simulink model "test"  (R2018a)
settings: Solver=VariableStepAuto  StartTime=0.0  StopTime=50  RelTol=1e-3
values from neighbouring files (symbols this model uses):
  A = [0 0 0 0 1 0 0 0 0 2.100456621 0 36.0401472471 ... (16 elements, 4x4)]    [optimal_a1.mat]    (also in optimal_a2.mat; optimal_b1.mat; optimal_c1.mat; optimal_c3.mat)
  B = [0 0.931879601156 0 2.82216717491]    [optimal_a1.mat]    (also in optimal_a2.mat; optimal_b1.mat; optimal_c1.mat; optimal_c3.mat)
  C = [1  0  0  0; 0  0  1  0]    [optimal_a1.mat]    (also in optimal_a2.mat; optimal_b1.mat; optimal_c1.mat; optimal_c3.mat)
  K = [0.1 0.550888453972 -27.6408063473 -4.60513234818]    [optimal_a1.mat]    (also in optimal_a2.mat = [0.4472135955 1.2428536758 -29.6950840953 -4.98636240184]; optimal_b1.mat = [0.316227766017 1.01615558831 -28.7702516875 -4.84272508365]; optimal_c1.mat = [31.6227766017 47.4701642792 -361.940883681 -31.457508206]; optimal_c3.mat = [0.0707106781187 0.453214488249 -27.0041075124 -4.5223617678)
  L = [37.9755841509  0.0115288283108; 360.356054275  2.87212240852; -0.0524370122115  38.0244158491; 0.754608556582  397.684084568]    [optimal_a1.mat]    (also in optimal_a2.mat; optimal_b1.mat; optimal_c1.mat; optimal_c3.mat)
settings Model: Creator=lizehua2  LastModifiedBy=lizehua2

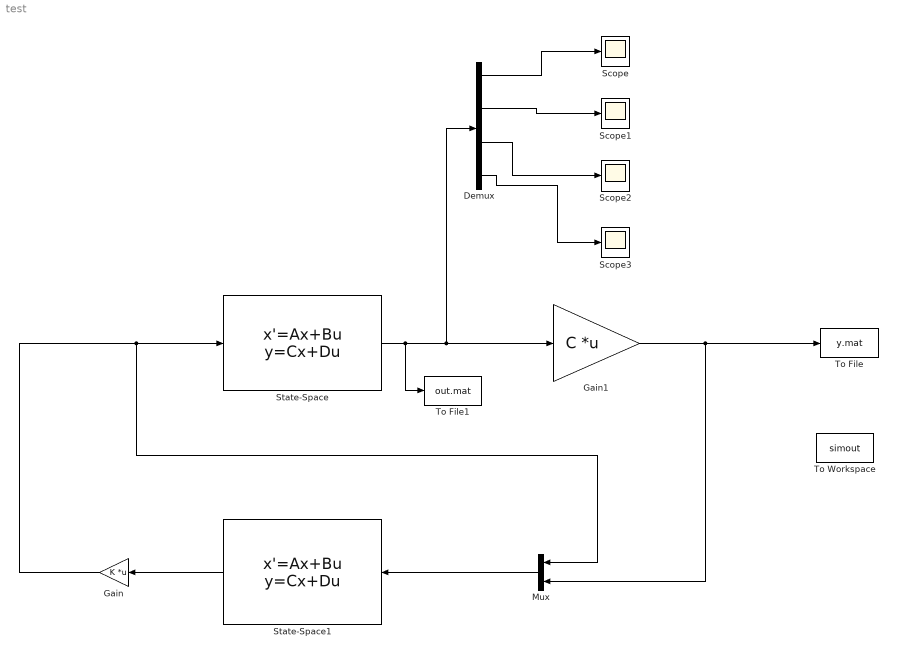
== system test ==
  Demux : Demux
  Gain : Gain  Gain=K  Multiplication=Matrix(K*u)
  Gain1 : Gain  Gain=C  Multiplication=Matrix(K*u)
  Mux : Mux  Inputs=2
  Scope{,1..3} (4 alike) : Scope
  State-Space : StateSpace  A=A  B=B  C=eye(4)  D=zeros(4,1)  InitialCondition=[0.5;0.1;0.175;0]
  State-Space1 : StateSpace  A=A-L*C  B=[B L]  C=eye(4)  D=zeros(4,3)  InitialCondition=[0.5;0.1;0.175;0]
  To File : ToFile  Filename=y.mat  MatrixName=y  SaveFormat=Timeseries
  To File1 : ToFile  Filename=out.mat  MatrixName=output
  To Workspace : ToWorkspace  VariableName=simout  SaveFormat=Timeseries  SampleTime=-1
  wires:
  State-Space1/1 -> Gain/1
  Gain/1 -> State-Space/1, Mux/1
  State-Space/1 -> To File1/1, Demux/1, Gain1/1
  Gain1/1 -> Mux/2, To File/1
  Mux/1 -> State-Space1/1
  Demux/1 -> Scope/1
  Demux/2 -> Scope1/1
  Demux/3 -> Scope2/1
  Demux/4 -> Scope3/1
